simulink model "es1_sim"  (Simulink 7.9)
settings: Solver=ode45  StartTime=0.0  StopTime=10.0  RelTol=1e-3
values from neighbouring files (symbols this model uses):
  A = [-7 -12;-1 -3]    [es1.m]
  B = [1 1]'    [es1.m]
  C = [1 1]    [es1.m]
  ueq = 2    [es1.m]
libraries: simulink x1
settings Model: Creator=patrizio  LastModifiedBy=patrizio
settings OptimizationCC: InlineInvariantSignals=on  InitFltsAndDblsToZero=on
settings DebuggingCC: SaveWithParameterizedLinksMsg=none  SignalResolutionControl=TryResolveAllWithWarning  MultiTaskDSMMsg=warning  MultiTaskCondExecSysMsg=none  StrictBusMsg=None
settings RTWCC: IncludeERTFirstTime=on
settings GRTTargetCC: TargetFcnLib=ansi_tfl_tmw.mat  CombineOutputUpdateFcns=off  GRTInterface=on

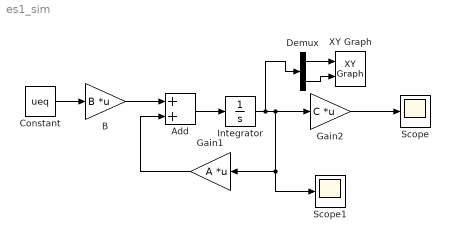
== system es1_sim ==
  Add : Sum
  B : Gain  Gain=B  Multiplication=Matrix(K*u)
  Constant : Constant  Value=ueq
  Demux : Demux  Outputs=2
  Gain1 : Gain  Gain=A  Multiplication=Matrix(K*u)
  Gain2 : Gain  Gain=C  Multiplication=Matrix(K*u)
  Integrator : Integrator
  Scope : Scope
  Scope1 : Scope
  XY Graph : simulink/Sinks/XY Graph  xmin=-1  xmax=1  ymin=-1  ymax=1  st=-1
  wires:
  Integrator/1 -> Gain2/1, Scope1/1, Gain1/1, Demux/1
  Add/1 -> Integrator/1
  B/1 -> Add/1
  Gain1/1 -> Add/2
  Constant/1 -> B/1
  Gain2/1 -> Scope/1
  Demux/1 -> XY Graph/1
  Demux/2 -> XY Graph/2
